simulink model "SF045A_HwAgSysArbn"  (R2013b)
settings: Solver=FixedStepDiscrete  SolverMode=SingleTasking  StartTime=0.0  StopTime=1  FixedStep=.002  RelTol=1e-3
values from neighbouring files (symbols this model uses):
  ARCHGLBPRM_2MILLISEC_SEC_F32 = DataDict.Constant    [SF045A_HwAgSysArbn_DataDict.m]
  CNVSECTOCNT_CNTPERSEC_U32 = DataDict.Constant    [SF045A_HwAgSysArbn_DataDict.m]
  CNVTOMILLISEC_MILLISECPERCNT_F32 = DataDict.Constant    [SF045A_HwAgSysArbn_DataDict.m]
  FltInj_f32 = DataDict.Client    [SF045A_HwAgSysArbn_DataDict.m]
  FLTINJ_HWAGSYSARBN_HWAG = DataDict.Constant    [SF045A_HwAgSysArbn_DataDict.m]
  FLTINJ_HWAGSYSARBN_SERLCOMHWAG = DataDict.Constant    [SF045A_HwAgSysArbn_DataDict.m]
  HwAgSysArbnHwAgConf1Snsr = DataDict.Calibration    [SF045A_HwAgSysArbn_DataDict.m]
  HwAgSysArbnHwAgConf2Snsr = DataDict.Calibration    [SF045A_HwAgSysArbn_DataDict.m]
  HwAgSysArbnHwAgConfNoSnsr = DataDict.Calibration    [SF045A_HwAgSysArbn_DataDict.m]
  HwAgSysArbnHwAgCorrdCorrlnThd = DataDict.Calibration    [SF045A_HwAgSysArbn_DataDict.m]
  HwAgSysArbnHwAgCorrlnFailDebStep = DataDict.Calibration    [SF045A_HwAgSysArbn_DataDict.m]
  HwAgSysArbnHwAgCorrlnPassDebStep = DataDict.Calibration    [SF045A_HwAgSysArbn_DataDict.m]
  HwAgSysArbnHwAgCorrlnRng = DataDict.Calibration    [SF045A_HwAgSysArbn_DataDict.m]
  HwAgSysArbnHwAgSlewRate = DataDict.Calibration    [SF045A_HwAgSysArbn_DataDict.m]
  HwAgSysArbnHwAgSnsrlsCorrlnThd = DataDict.Calibration    [SF045A_HwAgSysArbn_DataDict.m]
  HwAgSysArbnHwAgSnsrlsKineThd = DataDict.Calibration    [SF045A_HwAgSysArbn_DataDict.m]
  HwAgSysArbnHwAgToMotAgCorrlnElpdTiLim = DataDict.Calibration    [SF045A_HwAgSysArbn_DataDict.m]
  HwAgSysArbnSerlComHwAgCorrdConf = DataDict.Calibration    [SF045A_HwAgSysArbn_DataDict.m]
  HwAgSysArbnSerlComHwAgSnsrlsConf = DataDict.Calibration    [SF045A_HwAgSysArbn_DataDict.m]
  HwAgSysArbnSlewRateTmr = DataDict.Calibration    [SF045A_HwAgSysArbn_DataDict.m]
  HWAGTHD_ULS_FLOAT32 = DataDict.Constant    [SF045A_HwAgSysArbn_DataDict.m]
  INVLDSRC_CNT_S08 = DataDict.Constant    [SF045A_HwAgSysArbn_DataDict.m]
  LRGSLEW_HWDEGPERSEC_F32 = DataDict.Constant    [SF045A_HwAgSysArbn_DataDict.m]
  NODEBSTEP_CNT_U16 = DataDict.Constant    [SF045A_HwAgSysArbn_DataDict.m]
  SLEWINPROGS_CNT_LGC = DataDict.Constant    [SF045A_HwAgSysArbn_DataDict.m]
  SLEWNOTINPROGS_CNT_LGC = DataDict.Constant    [SF045A_HwAgSysArbn_DataDict.m]
  SNSRDATASRCSELD_CNT_S08 = DataDict.Constant    [SF045A_HwAgSysArbn_DataDict.m]
  SNSRLSDATASRCSELD_CNT_S08 = DataDict.Constant    [SF045A_HwAgSysArbn_DataDict.m]
  ZEROTMR_MILLISEC_F32 = DataDict.Constant    [SF045A_HwAgSysArbn_DataDict.m]
undefined symbols (not defined in the file or in its folder): NtcNr1, NtcSts1
libraries: simulink x10, NxtrLim x7, autosarlib x2, NxtrAbslt x2
(part 2 of 3)

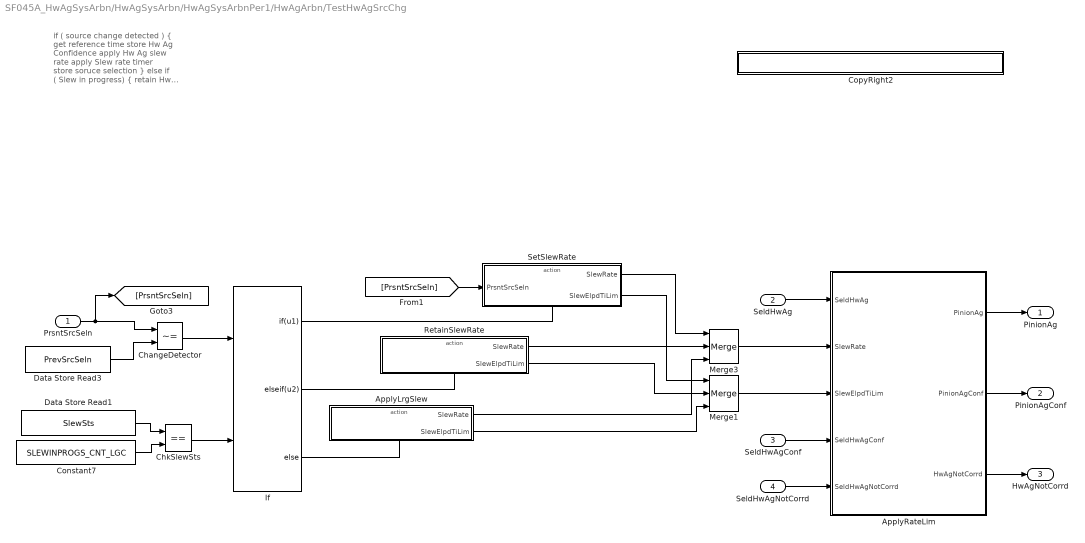
== system SF045A_HwAgSysArbn/HwAgSysArbn/HwAgSysArbnPer1/HwAgArbn/TestHwAgSrcChg ==
  note: if ( source change detected )
      | 	{
      |       get reference time
      |       store Hw Ag Confidence
      |       apply Hw Ag slew rate
      |       apply Slew rate timer
      |       store soruce selection
      | 	 }
      | else if ( Slew in progress)
      |      {
      |       retain Hw Ag slew rate
      |       retain Slew rate timer
      |       }
      |  else
      |    {
      |      apply large slew rate
      |      apply zero timer
      |     }
  PrsntSrcSeln : Inport
  SeldHwAg : Inport  Port=2
  SeldHwAgConf : Inport  Port=3
  SeldHwAgNotCorrd : Inport  Port=4
  " RetainSlewRate" : Subsystem  RequirementInfo={} %GIDa_cbbc3786_d9b6_473b_a98a_3e4d75800847  TreatAsAtomicUnit=on
  ApplyLrgSlew : Subsystem  TreatAsAtomicUnit=on
  ApplyRateLim : Subsystem
  ChangeDetector : RelationalOperator  RequirementInfo={} %GIDa_a662a9f5_a746_4973_9778_37a1843a9faa  Operator=~=  OutDataTypeStr=boolean
  ChkSlewSts : RelationalOperator  RequirementInfo={} %GIDa_1d9e48d6_a007_4919_9b9f_d83ebbd06af2  Operator===  OutDataTypeStr=boolean
  Constant7 : Constant  Value=SLEWINPROGS_CNT_LGC
  CopyRight2 : Subsystem  Description=|  mask(Copyright Information){none=on}
      | Copyright info block.                                               
      |                                                                     
      | Place copyright information at the top of every subsystem in design.
      mask prompts: none "No parameters"
      mask help: Place copyright information at the top of every subsystem in design.
      mask Display:
      | NxtrConf = 'Nexteer Confidential';
      | 
      | sys = bdroot; %handle for the current model ("system")
      | first = get_param(sys,'Created');
      | first = first(end-3:end);  %year is last four digits
      | 
      | last = get_param(sys,'LastModifiedDate');
      | if isempty(last)
      |     last = datestr(now,'yyyy');
      | else
      |     last = last(end-3:end);
      | end
      | 
      | if strcmp(first,last)
      |     fprintf('%s -- Copyright %s Nexteer',NxtrConf,first)
      | else
      |     fprintf('%s -- %s%s- %s Nexteer',NxtrConf,char(169),first,last)
      | end
  Data Store Read1 : DataStoreRead  RequirementInfo={} %GIDa_150ca47d_df79_478d_ac4a_7c7cb86a5ce2  DataStoreName=SlewSts
  Data Store Read3 : DataStoreRead  RequirementInfo={} %GIDa_8e5ad039_cbc9_4a86_8e5c_87b5b0910208  DataStoreName=PrevSrcSeln
  If : If  NumInputs=2  IfExpression=u1  ElseIfExpressions=u2
  Merge1 : Merge  Inputs=3
  Merge3 : Merge  Inputs=3
  SetSlewRate : Subsystem  RequirementInfo={} %GIDa_af6dfb04_f751_4e99_87d7_f680b57c5d18  TreatAsAtomicUnit=on
  PinionAg : Outport
  PinionAgConf : Outport  Port=2
  HwAgNotCorrd : Outport  Port=3
  wires:
  If/3 -> ApplyLrgSlew/Action
  SeldHwAg/1 -> ApplyRateLim/1(SeldHwAg)
  Merge3/1 -> ApplyRateLim/2(SlewRate)
  Merge1/1 -> ApplyRateLim/3(SlewElpdTiLim)
  ApplyRateLim/2(PinionAgConf) -> PinionAgConf/1
  ApplyRateLim/3(HwAgNotCorrd) -> HwAgNotCorrd/1
  ApplyRateLim/1(PinionAg) -> PinionAg/1
  SeldHwAgConf/1 -> ApplyRateLim/4(SeldHwAgConf)
  SeldHwAgNotCorrd/1 -> ApplyRateLim/5(SeldHwAgNotCorrd)
  If/1 -> SetSlewRate/Action
  If/2 -> " RetainSlewRate"/Action
  PrsntSrcSeln/1 -> ChangeDetector/1, [PrsntSrcSeln]
  Data Store Read3/1 -> ChangeDetector/2
  ChangeDetector/1 -> If/1
  [PrsntSrcSeln] -> SetSlewRate/1(PrsntSrcSeln)
  Data Store Read1/1 -> ChkSlewSts/1
  Constant7/1 -> ChkSlewSts/2
  ChkSlewSts/1 -> If/2
  SetSlewRate/1(SlewRate) -> Merge3/1
  " RetainSlewRate"/1(SlewRate) -> Merge3/2
  ApplyLrgSlew/2(SlewElpdTiLim) -> Merge1/3
  ApplyLrgSlew/1(SlewRate) -> Merge3/3
  SetSlewRate/2("SlewElpdTiLim ") -> Merge1/1
  " RetainSlewRate"/2("SlewElpdTiLim ") -> Merge1/2

== system SF045A_HwAgSysArbn/HwAgSysArbn/HwAgSysArbnPer1/HwAgArbn/VldtSnsrlsData ==
  HwAgSnsrlsIn : Inport
  HwAgSnsrlsConfIn : Inport  Port=2
  Abslt_f32_f1 : NxtrAbslt/Abslt_f32_f32  RequirementInfo={} %GIDa_5860b5a6_3a96_422b_aad5_4fb770ea0a9c  SFunctionSpec=single y1 = Abslt_f32_f32(single u1)
      settings: AttributesFormatString=%<Name>
  Constant7 : Constant  RequirementInfo={} %GIDa_bb195792_9ebd_40c7_985a_c670bff92963  Value=HwAgSysArbnHwAgSnsrlsKineThd
  CopyRight2 : Subsystem  Description=|  mask(Copyright Information){none=on}
      | Copyright info block.                                               
      |                                                                     
      | Place copyright information at the top of every subsystem in design.
      mask prompts: none "No parameters"
      mask help: Place copyright information at the top of every subsystem in design.
      mask Display:
      | NxtrConf = 'Nexteer Confidential';
      | 
      | sys = bdroot; %handle for the current model ("system")
      | first = get_param(sys,'Created');
      | first = first(end-3:end);  %year is last four digits
      | 
      | last = get_param(sys,'LastModifiedDate');
      | if isempty(last)
      |     last = datestr(now,'yyyy');
      | else
      |     last = last(end-3:end);
      | end
      | 
      | if strcmp(first,last)
      |     fprintf('%s -- Copyright %s Nexteer',NxtrConf,first)
      | else
      |     fprintf('%s -- %s%s- %s Nexteer',NxtrConf,char(169),first,last)
      | end
  Data Store Read2 : DataStoreRead  RequirementInfo={} %GIDa_545972b2_46c3_460d_a7e1_9bb6bef072c1  DataStoreName=HwAgKineFlt
  If : If  IfExpression=u1
  Logical Operator : Logic  Operator=NOT  AllPortsSameDT=off  OutDataTypeStr=boolean
  Logical Operator1 : Logic  AllPortsSameDT=off  OutDataTypeStr=boolean
  Merge1 : Merge
  Pass : Subsystem  TreatAsAtomicUnit=on
  Relational Operator4 : RelationalOperator  RequirementInfo={} %GIDa_3ef3c8f8_c499_409e_a413_21363b3c0e76  Operator=<=  OutDataTypeStr=boolean
  ThdExcdd : Subsystem  TreatAsAtomicUnit=on
  HwAgSnsrlsConf : Outport
  wires:
  Abslt_f32_f1/1 -> Relational Operator4/1
  ThdExcdd/1(Out) -> Merge1/2
  HwAgSnsrlsIn/1 -> Abslt_f32_f1/1
  Constant7/1 -> Relational Operator4/2
  If/1 -> Pass/Action
  If/2 -> ThdExcdd/Action
  Merge1/1 -> HwAgSnsrlsConf/1
  HwAgSnsrlsConfIn/1 -> Pass/1(In)
  Relational Operator4/1 -> Logical Operator1/1
  Data Store Read2/1 -> Logical Operator/1
  Logical Operator/1 -> Logical Operator1/2
  Logical Operator1/1 -> If/1
  Pass/1(Out) -> Merge1/1

== system SF045A_HwAgSysArbn/HwAgSysArbn/HwAgSysArbnInit1/Kinematic Integrity/SetNtcSts/CopyRight2 ==

== system SF045A_HwAgSysArbn/HwAgSysArbn/HwAgSysArbnPer1/FltInj_f32 client/CodeGen/CopyRight1 ==

== system SF045A_HwAgSysArbn/HwAgSysArbn/HwAgSysArbnPer1/FltInj_f32 client/Sim/CopyRight1 ==

== system SF045A_HwAgSysArbn/HwAgSysArbn/HwAgSysArbnPer1/FltInj_f32 client1/CodeGen/CopyRight1 ==

== system SF045A_HwAgSysArbn/HwAgSysArbn/HwAgSysArbnPer1/FltInj_f32 client1/Sim/CopyRight1 ==

== system SF045A_HwAgSysArbn/HwAgSysArbn/HwAgSysArbnPer1/HwAgArbn/CalcHwAgCorrdConf /CopyRight2 ==

== system SF045A_HwAgSysArbn/HwAgSysArbn/HwAgSysArbnPer1/HwAgArbn/CalcHwAgCorrdConf /NoSensor ==
  Action Port : ActionPort  ActionType=case
  Constant6 : Constant  RequirementInfo={} %GIDa_f14027cb_0e69_4f08_8bdf_1c2f91abdd8c  Value=HwAgSysArbnHwAgConfNoSnsr
  CopyRight2 : Subsystem  Description=|  mask(Copyright Information){none=on}
      | Copyright info block.                                               
      |                                                                     
      | Place copyright information at the top of every subsystem in design.
      mask prompts: none "No parameters"
      mask help: Place copyright information at the top of every subsystem in design.
      mask Display:
      | NxtrConf = 'Nexteer Confidential';
      | 
      | sys = bdroot; %handle for the current model ("system")
      | first = get_param(sys,'Created');
      | first = first(end-3:end);  %year is last four digits
      | 
      | last = get_param(sys,'LastModifiedDate');
      | if isempty(last)
      |     last = datestr(now,'yyyy');
      | else
      |     last = last(end-3:end);
      | end
      | 
      | if strcmp(first,last)
      |     fprintf('%s -- Copyright %s Nexteer',NxtrConf,first)
      | else
      |     fprintf('%s -- %s%s- %s Nexteer',NxtrConf,char(169),first,last)
      | end
  Out1 : Outport
  wires:
  Constant6/1 -> Out1/1

== system SF045A_HwAgSysArbn/HwAgSysArbn/HwAgSysArbnPer1/HwAgArbn/CalcHwAgCorrdConf /OneSensor ==
  Action Port : ActionPort  ActionType=case
  Constant6 : Constant  RequirementInfo={} %GIDa_9dadb87f_38de_4346_a930_d9cb3b8d21f4  Value=HwAgSysArbnHwAgConf1Snsr
  CopyRight2 : Subsystem  Description=|  mask(Copyright Information){none=on}
      | Copyright info block.                                               
      |                                                                     
      | Place copyright information at the top of every subsystem in design.
      mask prompts: none "No parameters"
      mask help: Place copyright information at the top of every subsystem in design.
      mask Display:
      | NxtrConf = 'Nexteer Confidential';
      | 
      | sys = bdroot; %handle for the current model ("system")
      | first = get_param(sys,'Created');
      | first = first(end-3:end);  %year is last four digits
      | 
      | last = get_param(sys,'LastModifiedDate');
      | if isempty(last)
      |     last = datestr(now,'yyyy');
      | else
      |     last = last(end-3:end);
      | end
      | 
      | if strcmp(first,last)
      |     fprintf('%s -- Copyright %s Nexteer',NxtrConf,first)
      | else
      |     fprintf('%s -- %s%s- %s Nexteer',NxtrConf,char(169),first,last)
      | end
  Out1 : Outport
  wires:
  Constant6/1 -> Out1/1

== system SF045A_HwAgSysArbn/HwAgSysArbn/HwAgSysArbnPer1/HwAgArbn/CalcHwAgCorrdConf /TwoSensors ==
  Action Port : ActionPort  ActionType=case
  Constant5 : Constant  RequirementInfo={} %GIDa_18ef479c_83d6_4a60_b32f_fd4ccc7fe2b5  Value=HwAgSysArbnHwAgConf2Snsr  OutDataTypeStr=single
      settings: AttributesFormatString=%<OutDataTypeStr>
  CopyRight2 : Subsystem  Description=|  mask(Copyright Information){none=on}
      | Copyright info block.                                               
      |                                                                     
      | Place copyright information at the top of every subsystem in design.
      mask prompts: none "No parameters"
      mask help: Place copyright information at the top of every subsystem in design.
      mask Display:
      | NxtrConf = 'Nexteer Confidential';
      | 
      | sys = bdroot; %handle for the current model ("system")
      | first = get_param(sys,'Created');
      | first = first(end-3:end);  %year is last four digits
      | 
      | last = get_param(sys,'LastModifiedDate');
      | if isempty(last)
      |     last = datestr(now,'yyyy');
      | else
      |     last = last(end-3:end);
      | end
      | 
      | if strcmp(first,last)
      |     fprintf('%s -- Copyright %s Nexteer',NxtrConf,first)
      | else
      |     fprintf('%s -- %s%s- %s Nexteer',NxtrConf,char(169),first,last)
      | end
  Out1 : Outport
  wires:
  Constant5/1 -> Out1/1

== system SF045A_HwAgSysArbn/HwAgSysArbn/HwAgSysArbnPer1/HwAgArbn/CalcHwAgCorrdConf /Zero ==
  Action Port : ActionPort  ActionType=default
  Constant5 : Constant  RequirementInfo={} %GIDa_26fc8475_3e7f_4f82_9a1f_7577f729359a  Value=0  OutDataTypeStr=single
      settings: AttributesFormatString=%<OutDataTypeStr>
  CopyRight2 : Subsystem  Description=|  mask(Copyright Information){none=on}
      | Copyright info block.                                               
      |                                                                     
      | Place copyright information at the top of every subsystem in design.
      mask prompts: none "No parameters"
      mask help: Place copyright information at the top of every subsystem in design.
      mask Display:
      | NxtrConf = 'Nexteer Confidential';
      | 
      | sys = bdroot; %handle for the current model ("system")
      | first = get_param(sys,'Created');
      | first = first(end-3:end);  %year is last four digits
      | 
      | last = get_param(sys,'LastModifiedDate');
      | if isempty(last)
      |     last = datestr(now,'yyyy');
      | else
      |     last = last(end-3:end);
      | end
      | 
      | if strcmp(first,last)
      |     fprintf('%s -- Copyright %s Nexteer',NxtrConf,first)
      | else
      |     fprintf('%s -- %s%s- %s Nexteer',NxtrConf,char(169),first,last)
      | end
  Out1 : Outport
  wires:
  Constant5/1 -> Out1/1

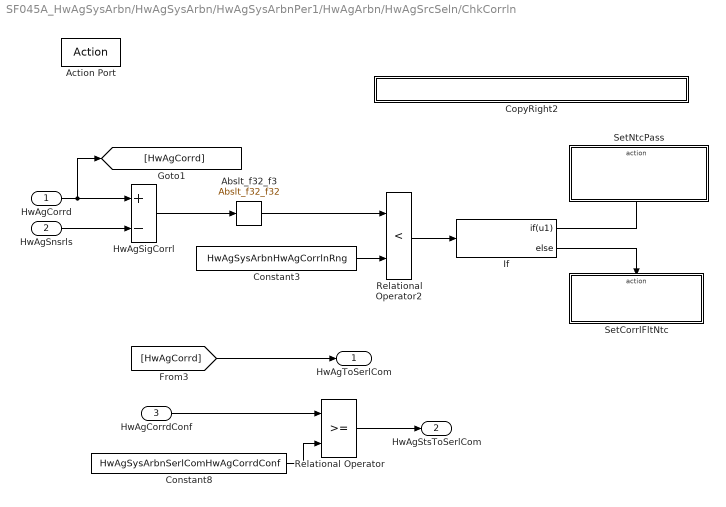
== system SF045A_HwAgSysArbn/HwAgSysArbn/HwAgSysArbnPer1/HwAgArbn/HwAgSrcSeln/ChkCorrln ==
  HwAgCorrd : Inport
  HwAgSnsrls : Inport  Port=2
  HwAgCorrdConf : Inport  Port=3
  Action Port : ActionPort  ActionType=then
  Abslt_f32_f3 : NxtrAbslt/Abslt_f32_f32  RequirementInfo={} %GIDa_77403248_8b35_41b2_902f_5d320c6d5c7c  SFunctionSpec=single y1 = Abslt_f32_f32(single u1)
      settings: AttributesFormatString=%<Name>
  Constant3 : Constant  RequirementInfo={} %GIDa_85c9f973_1d06_410f_8e8b_d947e0f9ea4c  Value=HwAgSysArbnHwAgCorrlnRng
  Constant8 : Constant  RequirementInfo={} %GIDa_c8ade5aa_b817_493c_9105_731119f5cd88  Value=HwAgSysArbnSerlComHwAgCorrdConf
  CopyRight2 : Subsystem  Description=|  mask(Copyright Information){none=on}
      | Copyright info block.                                               
      |                                                                     
      | Place copyright information at the top of every subsystem in design.
      mask prompts: none "No parameters"
      mask help: Place copyright information at the top of every subsystem in design.
      mask Display:
      | NxtrConf = 'Nexteer Confidential';
      | 
      | sys = bdroot; %handle for the current model ("system")
      | first = get_param(sys,'Created');
      | first = first(end-3:end);  %year is last four digits
      | 
      | last = get_param(sys,'LastModifiedDate');
      | if isempty(last)
      |     last = datestr(now,'yyyy');
      | else
      |     last = last(end-3:end);
      | end
      | 
      | if strcmp(first,last)
      |     fprintf('%s -- Copyright %s Nexteer',NxtrConf,first)
      | else
      |     fprintf('%s -- %s%s- %s Nexteer',NxtrConf,char(169),first,last)
      | end
  HwAgSigCorrl : Sum  RequirementInfo={} %GIDa_8e4dc380_878a_40bb_84db_d8426cd5bc38  Inputs=+-
  If : If  IfExpression=u1
  Relational Operator : RelationalOperator  RequirementInfo={} %GIDa_be6088f4_0bc5_4d1f_947a_e5979a469817  OutDataTypeStr=boolean
  Relational Operator2 : RelationalOperator  RequirementInfo={} %GIDa_4b6e8f32_90a5_4f1f_8c83_ee578fb98940  Operator=<  OutDataTypeStr=boolean
  SetCorrlFltNtc : Subsystem  TreatAsAtomicUnit=on
  SetNtcPass : Subsystem  TreatAsAtomicUnit=on
  HwAgToSerlCom : Outport
  HwAgStsToSerlCom : Outport  Port=2
  wires:
  Constant3/1 -> Relational Operator2/2
  Relational Operator2/1 -> If/1
  If/1 -> SetNtcPass/Action
  If/2 -> SetCorrlFltNtc/Action
  Abslt_f32_f3/1 -> Relational Operator2/1
  HwAgCorrd/1 -> [HwAgCorrd], HwAgSigCorrl/1
  HwAgSnsrls/1 -> HwAgSigCorrl/2
  HwAgSigCorrl/1 -> Abslt_f32_f3/1
  [HwAgCorrd] -> HwAgToSerlCom/1
  Constant8/1 -> Relational Operator/2
  Relational Operator/1 -> HwAgStsToSerlCom/1
  HwAgCorrdConf/1 -> Relational Operator/1

== system SF045A_HwAgSysArbn/HwAgSysArbn/HwAgSysArbnPer1/HwAgArbn/HwAgSrcSeln/CopyRight2 ==

== system SF045A_HwAgSysArbn/HwAgSysArbn/HwAgSysArbnPer1/HwAgArbn/HwAgSrcSeln/NoHwAgDataToSerlCom ==
  Action Port : ActionPort  ActionType=else
  Constant1 : Constant  RequirementInfo={} %GIDa_36596318_d44a_4d93_b3d5_4b0d9e7d2e9f  Value=0  OutDataTypeStr=single
      settings: AttributesFormatString=%<OutDataTypeStr>
  Constant3 : Constant  RequirementInfo={} %GIDa_ff53dfb1_0187_48ba_ada9_2388b0684dd6  Value=0  OutDataTypeStr=boolean
      settings: AttributesFormatString=%<OutDataTypeStr>
  Constant4 : Constant  RequirementInfo={} %GIDa_79664ab7_b2c1_4220_85dd_6c3aa80f2bed  Value=false  OutDataTypeStr=boolean
      settings: AttributesFormatString=%<OutDataTypeStr>
  CopyRight2 : Subsystem  Description=|  mask(Copyright Information){none=on}
      | Copyright info block.                                               
      |                                                                     
      | Place copyright information at the top of every subsystem in design.
      mask prompts: none "No parameters"
      mask help: Place copyright information at the top of every subsystem in design.
      mask Display:
      | NxtrConf = 'Nexteer Confidential';
      | 
      | sys = bdroot; %handle for the current model ("system")
      | first = get_param(sys,'Created');
      | first = first(end-3:end);  %year is last four digits
      | 
      | last = get_param(sys,'LastModifiedDate');
      | if isempty(last)
      |     last = datestr(now,'yyyy');
      | else
      |     last = last(end-3:end);
      | end
      | 
      | if strcmp(first,last)
      |     fprintf('%s -- Copyright %s Nexteer',NxtrConf,first)
      | else
      |     fprintf('%s -- %s%s- %s Nexteer',NxtrConf,char(169),first,last)
      | end
  Data Store Write1 : DataStoreWrite  RequirementInfo={} %GIDa_88767422_0782_4098_92aa_fdc1fbcd7e34  DataStoreName=HwAgToMotAgCorrln
  HwAgToSerlCom : Outport  RequirementInfo={} %GIDa_50f78f98_f9eb_4585_ab59_ac1656f8777f
  HwAgStsToSerlCom : Outport  RequirementInfo={} %GIDa_c1d6aa45_9827_4c64_b7e4_c3e1220e6ede  Port=2
  wires:
  Constant3/1 -> HwAgStsToSerlCom/1
  Constant1/1 -> HwAgToSerlCom/1
  Constant4/1 -> Data Store Write1/1

== system SF045A_HwAgSysArbn/HwAgSysArbn/HwAgSysArbnPer1/HwAgArbn/HwAgSrcSeln/SnsrDataToSerlCom ==
  HwAgCorrd : Inport
  HwAgCorrdConf : Inport  Port=2
  Action Port : ActionPort  ActionType=elseif
  Constant4 : Constant  RequirementInfo={} %GIDa_504c38a4_e9e3_4c56_9b31_a224c835fd7f  Value=false  OutDataTypeStr=boolean
      settings: AttributesFormatString=%<OutDataTypeStr>
  Constant8 : Constant  RequirementInfo={} %GIDa_c4b15b4c_45a2_43be_be9a_8e62c47dac96  Value=HwAgSysArbnSerlComHwAgCorrdConf
  CopyRight2 : Subsystem  Description=|  mask(Copyright Information){none=on}
      | Copyright info block.                                               
      |                                                                     
      | Place copyright information at the top of every subsystem in design.
      mask prompts: none "No parameters"
      mask help: Place copyright information at the top of every subsystem in design.
      mask Display:
      | NxtrConf = 'Nexteer Confidential';
      | 
      | sys = bdroot; %handle for the current model ("system")
      | first = get_param(sys,'Created');
      | first = first(end-3:end);  %year is last four digits
      | 
      | last = get_param(sys,'LastModifiedDate');
      | if isempty(last)
      |     last = datestr(now,'yyyy');
      | else
      |     last = last(end-3:end);
      | end
      | 
      | if strcmp(first,last)
      |     fprintf('%s -- Copyright %s Nexteer',NxtrConf,first)
      | else
      |     fprintf('%s -- %s%s- %s Nexteer',NxtrConf,char(169),first,last)
      | end
  Data Store Write1 : DataStoreWrite  RequirementInfo={} %GIDa_0e556bbd_3c5e_488a_8c66_652b80da9628  DataStoreName=HwAgToMotAgCorrln
  Relational Operator : RelationalOperator  RequirementInfo={} %GIDa_70ace2be_ed9e_4c57_b587_c6a833288725  OutDataTypeStr=boolean
  HwAgToSerlCom : Outport
  HwAgStsToSerlCom : Outport  Port=2
  wires:
  HwAgCorrd/1 -> HwAgToSerlCom/1
  Constant8/1 -> Relational Operator/2
  Relational Operator/1 -> HwAgStsToSerlCom/1
  HwAgCorrdConf/1 -> Relational Operator/1
  Constant4/1 -> Data Store Write1/1

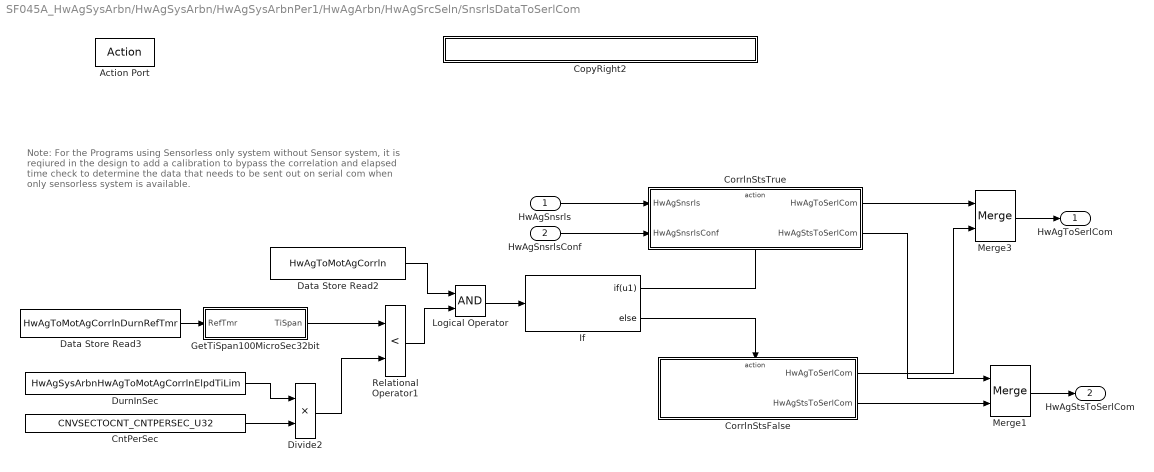
== system SF045A_HwAgSysArbn/HwAgSysArbn/HwAgSysArbnPer1/HwAgArbn/HwAgSrcSeln/SnsrlsDataToSerlCom ==
  note: Note: For the Programs using Sensorless only system without Sensor system,
      | it is reqiured in the design to add a calibration to bypass the correlation
      | and  elapsed time check to determine the data that needs to be
      | sent out on serial com when only sensorless system is available.
  HwAgSnsrls : Inport
  HwAgSnsrlsConf : Inport  Port=2
  Action Port : ActionPort  ActionType=elseif
  CntPerSec : Constant  RequirementInfo={} %GIDa_973e4c95_a2b8_4195_a681_0db90f1d458e  Value=CNVSECTOCNT_CNTPERSEC_U32
  CopyRight2 : Subsystem  Description=|  mask(Copyright Information){none=on}
      | Copyright info block.                                               
      |                                                                     
      | Place copyright information at the top of every subsystem in design.
      mask prompts: none "No parameters"
      mask help: Place copyright information at the top of every subsystem in design.
      mask Display:
      | NxtrConf = 'Nexteer Confidential';
      | 
      | sys = bdroot; %handle for the current model ("system")
      | first = get_param(sys,'Created');
      | first = first(end-3:end);  %year is last four digits
      | 
      | last = get_param(sys,'LastModifiedDate');
      | if isempty(last)
      |     last = datestr(now,'yyyy');
      | else
      |     last = last(end-3:end);
      | end
      | 
      | if strcmp(first,last)
      |     fprintf('%s -- Copyright %s Nexteer',NxtrConf,first)
      | else
      |     fprintf('%s -- %s%s- %s Nexteer',NxtrConf,char(169),first,last)
      | end
  CorrlnStsFalse : Subsystem  TreatAsAtomicUnit=on
  CorrlnStsTrue : Subsystem  TreatAsAtomicUnit=on
  Data Store Read2 : DataStoreRead  RequirementInfo={} %GIDa_da95b84a_e456_4838_818d_f36e6468da3b  DataStoreName=HwAgToMotAgCorrln
  Data Store Read3 : DataStoreRead  RequirementInfo={} %GIDa_b0225b62_f84f_4530_955c_c691a3cc05d0  DataStoreName=HwAgToMotAgCorrlnDurnRefTmr
  Divide2 : Product  RequirementInfo={} %GIDa_d722fcee_301b_44fa_b540_028c78ca9b46  Inputs=**
  DurnInSec : Constant  RequirementInfo={} %GIDa_5a8c34e4_0b9a_435d_b67f_8bfd191a712d  Value=HwAgSysArbnHwAgToMotAgCorrlnElpdTiLim
  GetTiSpan100MicroSec32bit : Subsystem  RequirementInfo={} %GIDa_12e04338_e781_4970_9e16_4bc87a3b1910
  If : If  IfExpression=u1
  Logical Operator : Logic  AllPortsSameDT=off  OutDataTypeStr=boolean
  Merge1 : Merge
  Merge3 : Merge
  Relational Operator1 : RelationalOperator  RequirementInfo={} %GIDa_b825364c_a1e4_4115_adc7_260db56aff26  Operator=<  OutDataTypeStr=boolean
  HwAgToSerlCom : Outport  RequirementInfo={} %GIDa_e87b3b32_bda8_40ab_a1c4_ede333da21e6
  HwAgStsToSerlCom : Outport  RequirementInfo={} %GIDa_6027c8a9_740c_4874_b9ce_764630c0e01f  Port=2
  wires:
  Logical Operator/1 -> If/1
  If/1 -> CorrlnStsTrue/Action
  If/2 -> CorrlnStsFalse/Action
  HwAgSnsrls/1 -> CorrlnStsTrue/1(HwAgSnsrls)
  HwAgSnsrlsConf/1 -> CorrlnStsTrue/2(HwAgSnsrlsConf)
  Merge1/1 -> HwAgStsToSerlCom/1
  Merge3/1 -> HwAgToSerlCom/1
  CorrlnStsFalse/1(HwAgToSerlCom) -> Merge3/2
  CorrlnStsFalse/2(HwAgStsToSerlCom) -> Merge1/2
  Relational Operator1/1 -> Logical Operator/2
  GetTiSpan100MicroSec32bit/1(TiSpan) -> Relational Operator1/1
  Divide2/1 -> Relational Operator1/2
  CntPerSec/1 -> Divide2/2
  Data Store Read2/1 -> Logical Operator/1
  Data Store Read3/1 -> GetTiSpan100MicroSec32bit/1(RefTmr)
  CorrlnStsTrue/1(HwAgToSerlCom) -> Merge3/1
  CorrlnStsTrue/2(HwAgStsToSerlCom) -> Merge1/1
  DurnInSec/1 -> Divide2/1

== system SF045A_HwAgSysArbn/HwAgSysArbn/HwAgSysArbnPer1/HwAgArbn/HwAgSrcSeln/SnsrlsHwAgSeln ==
  HwAgSnsrls : Inport
  HwAgSnsrlsConf : Inport  Port=2
  Action Port : ActionPort  ActionType=else
  CopyRight2 : Subsystem  Description=|  mask(Copyright Information){none=on}
      | Copyright info block.                                               
      |                                                                     
      | Place copyright information at the top of every subsystem in design.
      mask prompts: none "No parameters"
      mask help: Place copyright information at the top of every subsystem in design.
      mask Display:
      | NxtrConf = 'Nexteer Confidential';
      | 
      | sys = bdroot; %handle for the current model ("system")
      | first = get_param(sys,'Created');
      | first = first(end-3:end);  %year is last four digits
      | 
      | last = get_param(sys,'LastModifiedDate');
      | if isempty(last)
      |     last = datestr(now,'yyyy');
      | else
      |     last = last(end-3:end);
      | end
      | 
      | if strcmp(first,last)
      |     fprintf('%s -- Copyright %s Nexteer',NxtrConf,first)
      | else
      |     fprintf('%s -- %s%s- %s Nexteer',NxtrConf,char(169),first,last)
      | end
  SET : Constant  Value=SNSRLSDATASRCSELD_CNT_S08
  HwAgOut : Outport
  HwAgConfOut : Outport  Port=2
  HwAgNotCorrd : Outport  Port=3
  SrcSeln : Outport  Port=4
  wires:
  HwAgSnsrlsConf/1 -> HwAgConfOut/1
  HwAgSnsrls/1 -> HwAgNotCorrd/1, HwAgOut/1
  SET/1 -> SrcSeln/1

== system SF045A_HwAgSysArbn/HwAgSysArbn/HwAgSysArbnPer1/HwAgArbn/HwAgSrcSeln/VrfyHwAgCorrln ==
  HwAgCorrd : Inport
  HwAgCorrdConf : Inport  Port=2
  HwAg : Inport  Port=3
  Action Port : ActionPort  ActionType=then
  CopyRight2 : Subsystem  Description=|  mask(Copyright Information){none=on}
      | Copyright info block.                                               
      |                                                                     
      | Place copyright information at the top of every subsystem in design.
      mask prompts: none "No parameters"
      mask help: Place copyright information at the top of every subsystem in design.
      mask Display:
      | NxtrConf = 'Nexteer Confidential';
      | 
      | sys = bdroot; %handle for the current model ("system")
      | first = get_param(sys,'Created');
      | first = first(end-3:end);  %year is last four digits
      | 
      | last = get_param(sys,'LastModifiedDate');
      | if isempty(last)
      |     last = datestr(now,'yyyy');
      | else
      |     last = last(end-3:end);
      | end
      | 
      | if strcmp(first,last)
      |     fprintf('%s -- Copyright %s Nexteer',NxtrConf,first)
      | else
      |     fprintf('%s -- %s%s- %s Nexteer',NxtrConf,char(169),first,last)
      | end
  SET : Constant  Value=SNSRDATASRCSELD_CNT_S08
  HwAgOut : Outport
  HwAgConfOut : Outport  Port=2
  "HwAgNotCorrd " : Outport  Port=3
  SrcSeln : Outport  Port=4
  wires:
  HwAgCorrd/1 -> HwAgOut/1
  HwAgCorrdConf/1 -> HwAgConfOut/1
  HwAg/1 -> "HwAgNotCorrd "/1
  SET/1 -> SrcSeln/1

== system SF045A_HwAgSysArbn/HwAgSysArbn/HwAgSysArbnPer1/HwAgArbn/TestHwAgSrcChg/ RetainSlewRate ==
  Action Port : ActionPort  ActionType=elseif
  Constant2 : Constant  RequirementInfo={} %GIDa_204a868e_3f1d_4240_ac5a_180520e40449  Value=HwAgSysArbnHwAgSlewRate
  Constant4 : Constant  RequirementInfo={} %GIDa_3427d327_1b5d_4bda_aefd_4b15686addad  Value=HwAgSysArbnSlewRateTmr
  CopyRight2 : Subsystem  Description=|  mask(Copyright Information){none=on}
      | Copyright info block.                                               
      |                                                                     
      | Place copyright information at the top of every subsystem in design.
      mask prompts: none "No parameters"
      mask help: Place copyright information at the top of every subsystem in design.
      mask Display:
      | NxtrConf = 'Nexteer Confidential';
      | 
      | sys = bdroot; %handle for the current model ("system")
      | first = get_param(sys,'Created');
      | first = first(end-3:end);  %year is last four digits
      | 
      | last = get_param(sys,'LastModifiedDate');
      | if isempty(last)
      |     last = datestr(now,'yyyy');
      | else
      |     last = last(end-3:end);
      | end
      | 
      | if strcmp(first,last)
      |     fprintf('%s -- Copyright %s Nexteer',NxtrConf,first)
      | else
      |     fprintf('%s -- %s%s- %s Nexteer',NxtrConf,char(169),first,last)
      | end
  SlewRate : Outport
  "SlewElpdTiLim " : Outport  Port=2
  wires:
  Constant4/1 -> "SlewElpdTiLim "/1
  Constant2/1 -> SlewRate/1

== system SF045A_HwAgSysArbn/HwAgSysArbn/HwAgSysArbnPer1/HwAgArbn/TestHwAgSrcChg/ApplyLrgSlew ==
  Action Port : ActionPort  ActionType=else
  Constant1 : Constant  Value=LRGSLEW_HWDEGPERSEC_F32
  Constant3 : Constant  Value=ZEROTMR_MILLISEC_F32
  CopyRight2 : Subsystem  Description=|  mask(Copyright Information){none=on}
      | Copyright info block.                                               
      |                                                                     
      | Place copyright information at the top of every subsystem in design.
      mask prompts: none "No parameters"
      mask help: Place copyright information at the top of every subsystem in design.
      mask Display:
      | NxtrConf = 'Nexteer Confidential';
      | 
      | sys = bdroot; %handle for the current model ("system")
      | first = get_param(sys,'Created');
      | first = first(end-3:end);  %year is last four digits
      | 
      | last = get_param(sys,'LastModifiedDate');
      | if isempty(last)
      |     last = datestr(now,'yyyy');
      | else
      |     last = last(end-3:end);
      | end
      | 
      | if strcmp(first,last)
      |     fprintf('%s -- Copyright %s Nexteer',NxtrConf,first)
      | else
      |     fprintf('%s -- %s%s- %s Nexteer',NxtrConf,char(169),first,last)
      | end
  SlewRate : Outport
  SlewElpdTiLim : Outport  Port=2
  wires:
  Constant1/1 -> SlewRate/1
  Constant3/1 -> SlewElpdTiLim/1

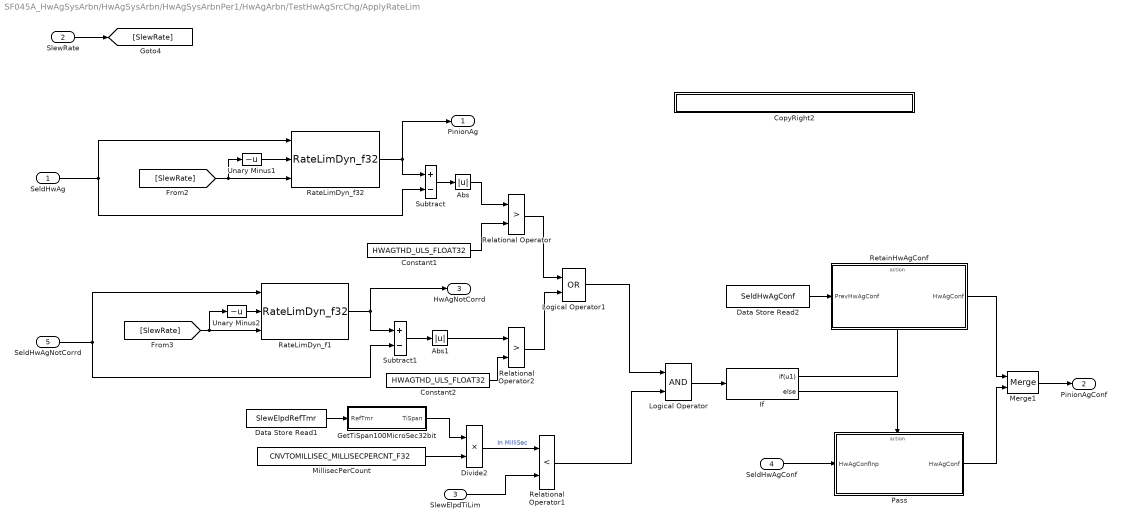
== system SF045A_HwAgSysArbn/HwAgSysArbn/HwAgSysArbnPer1/HwAgArbn/TestHwAgSrcChg/ApplyRateLim ==
  SeldHwAg : Inport  RequirementInfo={} %GIDa_47c3820a_94a9_49e9_ab3d_1467fef631cc
  SlewRate : Inport  RequirementInfo={} %GIDa_af9888fd_9c3a_4dad_a956_cca071cda959  Port=2
  SlewElpdTiLim : Inport  RequirementInfo={} %GIDa_8d81ebaa_bbde_485d_a47b_ee03bc18b359  Port=3
  SeldHwAgConf : Inport  Port=4
  SeldHwAgNotCorrd : Inport  RequirementInfo={} %GIDa_6d0620d6_e805_4d64_a3a8_51eb36635a4b  Port=5
  " RetainHwAgConf" : Subsystem  RequirementInfo={} %GIDa_4b3c3953_b3df_4b09_8079_ff55b3ce84b4  TreatAsAtomicUnit=on
  Abs : Abs  RequirementInfo={} %GIDa_ba368e3d_16a3_4b46_ba77_a04c6aa40b1b
  Abs1 : Abs  RequirementInfo={} %GIDa_9147af30_4419_451c_810b_23b571ca4024
  Constant1 : Constant  RequirementInfo={} %GIDa_cbe0846e_6f56_47da_9094_6fce400d2a9e  Value=HWAGTHD_ULS_FLOAT32
  Constant2 : Constant  RequirementInfo={} %GIDa_b5c3897b_0bdc_4ea6_8a24_bc2e51770e88  Value=HWAGTHD_ULS_FLOAT32
  CopyRight2 : Subsystem  Description=|  mask(Copyright Information){none=on}
      | Copyright info block.                                               
      |                                                                     
      | Place copyright information at the top of every subsystem in design.
      mask prompts: none "No parameters"
      mask help: Place copyright information at the top of every subsystem in design.
      mask Display:
      | NxtrConf = 'Nexteer Confidential';
      | 
      | sys = bdroot; %handle for the current model ("system")
      | first = get_param(sys,'Created');
      | first = first(end-3:end);  %year is last four digits
      | 
      | last = get_param(sys,'LastModifiedDate');
      | if isempty(last)
      |     last = datestr(now,'yyyy');
      | else
      |     last = last(end-3:end);
      | end
      | 
      | if strcmp(first,last)
      |     fprintf('%s -- Copyright %s Nexteer',NxtrConf,first)
      | else
      |     fprintf('%s -- %s%s- %s Nexteer',NxtrConf,char(169),first,last)
      | end
  Data Store Read1 : DataStoreRead  RequirementInfo={} %GIDa_a244de5b_8272_4cde_9f73_f7329a068225  DataStoreName=SlewElpdRefTmr
  Data Store Read2 : DataStoreRead  RequirementInfo={} %GIDa_f5fb1cf9_86e8_4a7e_aa1c_254981741c40  DataStoreName=SeldHwAgConf
  Divide2 : Product  RequirementInfo={} %GIDa_2709fbe9_e04d_4ee8_bf50_5d60d9575a78  Inputs=**
  GetTiSpan100MicroSec32bit : Subsystem  RequirementInfo={} %GIDa_1d40f879_b9a1_49bd_9e5b_06c72c99222f
  If : If  IfExpression=u1
  Logical Operator : Logic  RequirementInfo={} %GIDa_b1fcbfac_aa09_4583_9e54_60d53ca1f970  AllPortsSameDT=off  OutDataTypeStr=boolean
  Logical Operator1 : Logic  RequirementInfo={} %GIDa_2025a4cc_5d44_45bd_b6bf_4612c0b4b1eb  Operator=OR  AllPortsSameDT=off  OutDataTypeStr=boolean
  Merge1 : Merge
  MillisecPerCount : Constant  RequirementInfo={} %GIDa_019366f1_44f7_4d8a_bfcf_6b9c8a926f2e  Value=CNVTOMILLISEC_MILLISECPERCNT_F32
  Pass : Subsystem  TreatAsAtomicUnit=on
  RateLimDyn_f1 : NxtrLim/RateLimDyn_f32  RequirementInfo={} %GIDa_59329933_5b08_48b2_abba_1a876b5f738c  StVar=PrevHwAgNotCorrd  Ts=ARCHGLBPRM_2MILLISEC_SEC_F32
      settings: AttributesFormatString=StVar: %<StVar>
  RateLimDyn_f32 : NxtrLim/RateLimDyn_f32  RequirementInfo={} %GIDa_88d4e2a4_e592_4202_9a3b_8e94e50a8167  StVar=PrevSeldHwAg  Ts=ARCHGLBPRM_2MILLISEC_SEC_F32
      settings: AttributesFormatString=StVar: %<StVar>
  Relational Operator : RelationalOperator  RequirementInfo={} %GIDa_3f5c862c_62c2_42f7_851b_c88d52ef0bec  Operator=>  OutDataTypeStr=boolean
  Relational Operator1 : RelationalOperator  RequirementInfo={} %GIDa_8dea15be_a1b5_405c_9a92_47e8aa1d57cc  Operator=<  OutDataTypeStr=boolean
  Relational Operator2 : RelationalOperator  RequirementInfo={} %GIDa_d82b9e5e_368e_4148_acc2_adf54ff462a3  Operator=>  OutDataTypeStr=boolean
  Subtract : Sum  RequirementInfo={} %GIDa_cc8579d9_7186_4802_ba2e_856045be2b03  Inputs=+-
  Subtract1 : Sum  RequirementInfo={} %GIDa_b662939e_2ab2_4b65_946f_061900322dfd  Inputs=+-
  Unary Minus1 : UnaryMinus  RequirementInfo={} %GIDa_8f1614a8_f49f_44ad_b0e0_242b260b3df6
  Unary Minus2 : UnaryMinus  RequirementInfo={} %GIDa_a4f1d02c_67ef_441a_9b4d_93283f796036
  PinionAg : Outport  RequirementInfo={} %GIDa_2088590c_22d0_4df1_8099_800edad66be5
  PinionAgConf : Outport  Port=2
  HwAgNotCorrd : Outport  RequirementInfo={} %GIDa_b98fdcca_b0dd_40f4_9b0c_a717bdab7737  Port=3
  wires:
  SeldHwAg/1 -> Subtract/2, RateLimDyn_f32/1
  [SlewRate] -> Unary Minus1/1, RateLimDyn_f32/3
  Unary Minus1/1 -> RateLimDyn_f32/2
  Subtract/1 -> Abs/1
  Abs/1 -> Relational Operator/1
  Constant1/1 -> Relational Operator/2
  Relational Operator1/1 -> Logical Operator/2
  Logical Operator/1 -> If/1
  If/1 -> " RetainHwAgConf"/Action
  If/2 -> Pass/Action
  Data Store Read2/1 -> " RetainHwAgConf"/1(PrevHwAgConf)
  SeldHwAgConf/1 -> Pass/1(HwAgConfInp)
  Merge1/1 -> PinionAgConf/1
  " RetainHwAgConf"/1("HwAgConf ") -> Merge1/1
  Pass/1("HwAgConf ") -> Merge1/2
  Divide2/1 -> Relational Operator1/1  "In MilliSec"
  SlewElpdTiLim/1 -> Relational Operator1/2
  Data Store Read1/1 -> GetTiSpan100MicroSec32bit/1(RefTmr)
  RateLimDyn_f32/1 -> PinionAg/1, Subtract/1
  GetTiSpan100MicroSec32bit/1(TiSpan) -> Divide2/1
  MillisecPerCount/1 -> Divide2/2
  SlewRate/1 -> [SlewRate]
  [SlewRate] -> Unary Minus2/1, RateLimDyn_f1/3
  Unary Minus2/1 -> RateLimDyn_f1/2
  SeldHwAgNotCorrd/1 -> Subtract1/2, RateLimDyn_f1/1
  Subtract1/1 -> Abs1/1
  Abs1/1 -> Relational Operator2/1
  Constant2/1 -> Relational Operator2/2
  RateLimDyn_f1/1 -> HwAgNotCorrd/1, Subtract1/1
  Relational Operator/1 -> Logical Operator1/1
  Relational Operator2/1 -> Logical Operator1/2
  Logical Operator1/1 -> Logical Operator/1

== system SF045A_HwAgSysArbn/HwAgSysArbn/HwAgSysArbnPer1/HwAgArbn/TestHwAgSrcChg/CopyRight2 ==

== system SF045A_HwAgSysArbn/HwAgSysArbn/HwAgSysArbnPer1/HwAgArbn/TestHwAgSrcChg/SetSlewRate ==
  PrsntSrcSeln : Inport  RequirementInfo={} %GIDa_81b7eb70_73b5_43dd_8a28_bb224dded635
  Action Port : ActionPort  ActionType=then
  Constant5 : Constant  RequirementInfo={} %GIDa_10659385_b7e2_489a_9dfc_cb6f7067b33d  Value=HwAgSysArbnHwAgSlewRate
  Constant6 : Constant  RequirementInfo={} %GIDa_378a5a7e_5466_4899_a26f_200ebd38aedc  Value=HwAgSysArbnSlewRateTmr
  CopyRight2 : Subsystem  Description=|  mask(Copyright Information){none=on}
      | Copyright info block.                                               
      |                                                                     
      | Place copyright information at the top of every subsystem in design.
      mask prompts: none "No parameters"
      mask help: Place copyright information at the top of every subsystem in design.
      mask Display:
      | NxtrConf = 'Nexteer Confidential';
      | 
      | sys = bdroot; %handle for the current model ("system")
      | first = get_param(sys,'Created');
      | first = first(end-3:end);  %year is last four digits
      | 
      | last = get_param(sys,'LastModifiedDate');
      | if isempty(last)
      |     last = datestr(now,'yyyy');
      | else
      |     last = last(end-3:end);
      | end
      | 
      | if strcmp(first,last)
      |     fprintf('%s -- Copyright %s Nexteer',NxtrConf,first)
      | else
      |     fprintf('%s -- %s%s- %s Nexteer',NxtrConf,char(169),first,last)
      | end
  Data Store Read2 : DataStoreRead  RequirementInfo={} %GIDa_fd01000c_a5a4_4f03_8777_94812053c236  DataStoreName=PrevPinionAgConf
  Data Store Write2 : DataStoreWrite  RequirementInfo={} %GIDa_b8863701_8dbf_443d_abc7_a04d9d557b14  DataStoreName=SeldHwAgConf
  Data Store Write3 : DataStoreWrite  RequirementInfo={} %GIDa_eb32eb1d_3507_4b21_9798_4cc8c1f1e2f2  DataStoreName=SlewElpdRefTmr
  Data Store Write6 : DataStoreWrite  RequirementInfo={} %GIDa_4f1741a0_d6b1_46a7_b6f2_4a887c2fe202  DataStoreName=PrevSrcSeln
  GetRefTmr100MicroSec32bit : Subsystem  RequirementInfo={} %GIDa_280f004b_76c5_474d_b09f_1cecc41ed2e8
  SlewRate : Outport
  "SlewElpdTiLim " : Outport  Port=2
  wires:
  Data Store Read2/1 -> Data Store Write2/1
  PrsntSrcSeln/1 -> Data Store Write6/1
  GetRefTmr100MicroSec32bit/1(RefTmr) -> Data Store Write3/1
  Constant5/1 -> SlewRate/1
  Constant6/1 -> "SlewElpdTiLim "/1

== system SF045A_HwAgSysArbn/HwAgSysArbn/HwAgSysArbnPer1/HwAgArbn/VldtSnsrlsData/CopyRight2 ==

== system SF045A_HwAgSysArbn/HwAgSysArbn/HwAgSysArbnPer1/HwAgArbn/VldtSnsrlsData/Pass ==
  In : Inport
  Action Port : ActionPort  ActionType=then
  CopyRight2 : Subsystem  Description=|  mask(Copyright Information){none=on}
      | Copyright info block.                                               
      |                                                                     
      | Place copyright information at the top of every subsystem in design.
      mask prompts: none "No parameters"
      mask help: Place copyright information at the top of every subsystem in design.
      mask Display:
      | NxtrConf = 'Nexteer Confidential';
      | 
      | sys = bdroot; %handle for the current model ("system")
      | first = get_param(sys,'Created');
      | first = first(end-3:end);  %year is last four digits
      | 
      | last = get_param(sys,'LastModifiedDate');
      | if isempty(last)
      |     last = datestr(now,'yyyy');
      | else
      |     last = last(end-3:end);
      | end
      | 
      | if strcmp(first,last)
      |     fprintf('%s -- Copyright %s Nexteer',NxtrConf,first)
      | else
      |     fprintf('%s -- %s%s- %s Nexteer',NxtrConf,char(169),first,last)
      | end
  Out : Outport
  wires:
  In/1 -> Out/1

== system SF045A_HwAgSysArbn/HwAgSysArbn/HwAgSysArbnPer1/HwAgArbn/VldtSnsrlsData/ThdExcdd ==
  Action Port : ActionPort  ActionType=else
  Constant1 : Constant  RequirementInfo={} %GIDa_00df5f9f_69ae_4346_a770_c7586c4ead39  Value=0
  Constant2 : Constant  RequirementInfo={} %GIDa_36b8a02b_dfe2_42c0_a30d_d97766948556  Value=NODEBSTEP_CNT_U16
  CopyRight2 : Subsystem  Description=|  mask(Copyright Information){none=on}
      | Copyright info block.                                               
      |                                                                     
      | Place copyright information at the top of every subsystem in design.
      mask prompts: none "No parameters"
      mask help: Place copyright information at the top of every subsystem in design.
      mask Display:
      | NxtrConf = 'Nexteer Confidential';
      | 
      | sys = bdroot; %handle for the current model ("system")
      | first = get_param(sys,'Created');
      | first = first(end-3:end);  %year is last four digits
      | 
      | last = get_param(sys,'LastModifiedDate');
      | if isempty(last)
      |     last = datestr(now,'yyyy');
      | else
      |     last = last(end-3:end);
      | end
      | 
      | if strcmp(first,last)
      |     fprintf('%s -- Copyright %s Nexteer',NxtrConf,first)
      | else
      |     fprintf('%s -- %s%s- %s Nexteer',NxtrConf,char(169),first,last)
      | end
  Data Store Write3 : DataStoreWrite  RequirementInfo={} %GIDa_0732693a_f875_4b62_9c7d_a331460b0957  DataStoreName=HwAgKineFlt
  Enumerated Constant1 : simulink/Sources/Enumerated Constant  RequirementInfo={} %GIDa_7b1db603_75d5_4653_a78d_f670211fc6f8  OutDataTypeStr=Enum: NtcSts1  Value=NtcSts1.NTCSTS_FAILD  SampleTime=inf
  Enumerated Constant2 : simulink/Sources/Enumerated Constant  RequirementInfo={} %GIDa_09b65c6b_ffa2_466b_8bb2_d6db1aa6db3d  OutDataTypeStr=Enum: NtcNr1  Value=NtcNr1.NTCNR_0X0A1  SampleTime=inf
  Kinematic Integrity : Subsystem  RequirementInfo={} %GIDa_58808720_4ea4_4840_aab3_60d84eff6aaf  mask(SetNTC){}
      mask help: SetNTC library block
  SET1 : Constant  Value=0  OutDataTypeStr=single
      settings: AttributesFormatString=%<OutDataTypeStr>
  SET2 : Constant  Value=true  OutDataTypeStr=boolean
      settings: AttributesFormatString=%<OutDataTypeStr>
  Out : Outport
  wires:
  Enumerated Constant1/1 -> Kinematic Integrity/3(NtcSts)
  Constant1/1 -> Kinematic Integrity/2(NtcStInfo)
  Enumerated Constant2/1 -> Kinematic Integrity/1(NtcNr)
  Constant2/1 -> Kinematic Integrity/4(DebStep)
  SET1/1 -> Out/1
  SET2/1 -> Data Store Write3/1

== system SF045A_HwAgSysArbn/HwAgSysArbn/HwAgSysArbnPer1/HwAgArbn/CalcHwAgCorrdConf /NoSensor/CopyRight2 ==

== system SF045A_HwAgSysArbn/HwAgSysArbn/HwAgSysArbnPer1/HwAgArbn/CalcHwAgCorrdConf /OneSensor/CopyRight2 ==

== system SF045A_HwAgSysArbn/HwAgSysArbn/HwAgSysArbnPer1/HwAgArbn/CalcHwAgCorrdConf /TwoSensors/CopyRight2 ==

== system SF045A_HwAgSysArbn/HwAgSysArbn/HwAgSysArbnPer1/HwAgArbn/CalcHwAgCorrdConf /Zero/CopyRight2 ==

== system SF045A_HwAgSysArbn/HwAgSysArbn/HwAgSysArbnPer1/HwAgArbn/HwAgSrcSeln/ChkCorrln/CopyRight2 ==

== system SF045A_HwAgSysArbn/HwAgSysArbn/HwAgSysArbnPer1/HwAgArbn/HwAgSrcSeln/ChkCorrln/SetCorrlFltNtc ==
  Action Port : ActionPort  ActionType=else
  Constant1 : Constant  RequirementInfo={} %GIDa_bd9bbf13_b56c_4d7e_8c7b_cd5cc212371e  Value=0
  Constant2 : Constant  RequirementInfo={} %GIDa_3683a39a_4af4_45fd_aee7_cbcaac274b79  Value=HwAgSysArbnHwAgCorrlnFailDebStep
  Constant4 : Constant  RequirementInfo={} %GIDa_9cdf1038_f771_410f_a05a_803482fb4a33  Value=false  OutDataTypeStr=boolean
      settings: AttributesFormatString=%<OutDataTypeStr>
  CopyRight2 : Subsystem  Description=|  mask(Copyright Information){none=on}
      | Copyright info block.                                               
      |                                                                     
      | Place copyright information at the top of every subsystem in design.
      mask prompts: none "No parameters"
      mask help: Place copyright information at the top of every subsystem in design.
      mask Display:
      | NxtrConf = 'Nexteer Confidential';
      | 
      | sys = bdroot; %handle for the current model ("system")
      | first = get_param(sys,'Created');
      | first = first(end-3:end);  %year is last four digits
      | 
      | last = get_param(sys,'LastModifiedDate');
      | if isempty(last)
      |     last = datestr(now,'yyyy');
      | else
      |     last = last(end-3:end);
      | end
      | 
      | if strcmp(first,last)
      |     fprintf('%s -- Copyright %s Nexteer',NxtrConf,first)
      | else
      |     fprintf('%s -- %s%s- %s Nexteer',NxtrConf,char(169),first,last)
      | end
  Data Store Write1 : DataStoreWrite  RequirementInfo={} %GIDa_8f5b8848_57bf_42e5_9e9f_ca406721d3a2  DataStoreName=HwAgToMotAgCorrln
  Enumerated Constant1 : simulink/Sources/Enumerated Constant  RequirementInfo={} %GIDa_32b2a30c_7348_49dd_81d9_88b6d1b3e356  OutDataTypeStr=Enum: NtcSts1  Value=NtcSts1.NTCSTS_PREFAILD  SampleTime=inf
  Enumerated Constant15 : simulink/Sources/Enumerated Constant  RequirementInfo={} %GIDa_193d95fa_ac48_45c6_a9f9_8c411be8b224  OutDataTypeStr=Enum: NtcNr1  Value=NtcNr1.NTCNR_0X0A6  SampleTime=inf
  SetCorrlFltNtc : Subsystem  RequirementInfo={} %GIDa_f7296c4d_77d3_4204_8281_53acb2ecd210  mask(SetNTC){}
      mask help: SetNTC library block
  wires:
  Enumerated Constant1/1 -> SetCorrlFltNtc/3(NtcSts)
  Constant1/1 -> SetCorrlFltNtc/2(NtcStInfo)
  Enumerated Constant15/1 -> SetCorrlFltNtc/1(NtcNr)
  Constant2/1 -> SetCorrlFltNtc/4(DebStep)
  Constant4/1 -> Data Store Write1/1
